simulink model "nonlinearpendulum"  (R2023b)
settings: Solver=VariableStepAuto  StartTime=0.0  StopTime=10.0  RelTol=1e-3
values from neighbouring files (symbols this model uses):
  g = 10    [non_linear_pendulum_0611.m]
  l = 1    [non_linear_pendulum_0611.m]
  m = 1    [non_linear_pendulum_0611.m]
  Teq = 0    [non_linear_pendulum_0611.m]
settings Model: Creator=martinhaugen  LastModifiedBy=martinhaugen

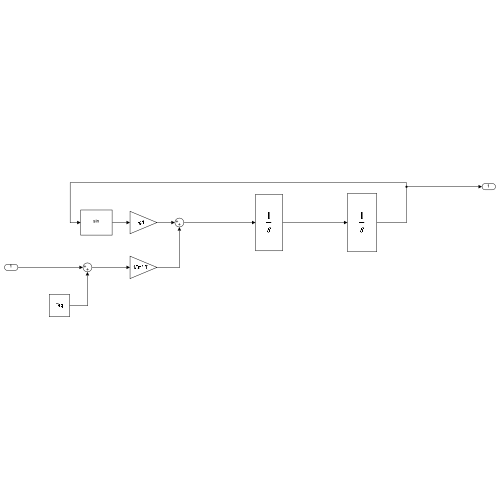
[thumbnail: Simulink's stored preview of the top-level diagram]
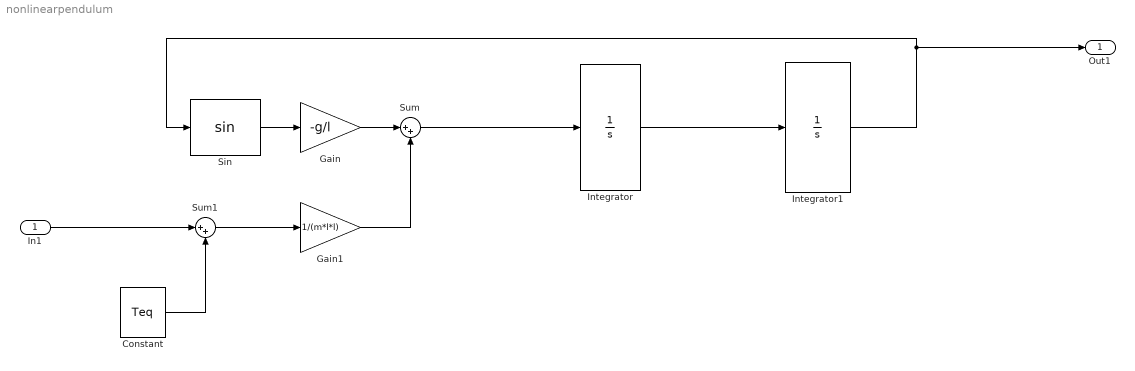
== system nonlinearpendulum ==
  In1 : Inport
  Constant : Constant  Value=Teq
  Gain : Gain  Gain=-g/l
  Gain1 : Gain  Gain=1/(m*l*l)
  Integrator : Integrator
  Integrator1 : Integrator
  Sin : Trigonometry
  Sum : Sum  Inputs=|++
  Sum1 : Sum  Inputs=|++
  Out1 : Outport
  wires:
  Sum/1 -> Integrator/1
  Integrator/1 -> Integrator1/1
  Sin/1 -> Gain/1
  Gain/1 -> Sum/1
  In1/1 -> Sum1/1
  Gain1/1 -> Sum/2
  Integrator1/1 -> Out1/1, Sin/1
  Constant/1 -> Sum1/2
  Sum1/1 -> Gain1/1
